simulink model "Activity_8"  (R2019b)
settings: Solver=VariableStepAuto  StartTime=0.0  StopTime=0.002  RelTol=1e-3
libraries: dspsrcs4 x3, dspfdesign x1
settings Model: Creator=linesLK  LastModifiedBy=linesLK

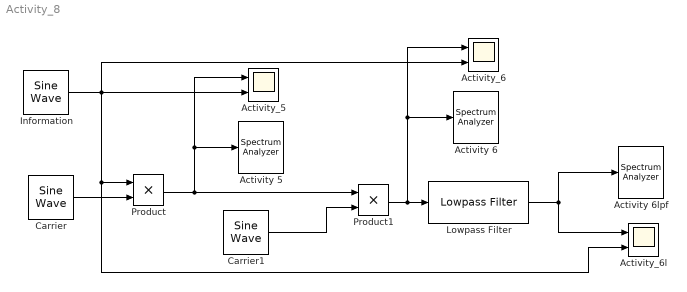
== system Activity_8 ==
  Activity 5 : SpectrumAnalyzer
  Activity 6 : SpectrumAnalyzer
  Activity 6lpf : SpectrumAnalyzer
  Activity_5 : Scope  NumInputPorts=2
  Activity_6 : Scope  NumInputPorts=2
  Activity_6l : Scope  NumInputPorts=2
  Carrier : dspsrcs4/Sine Wave  Amplitude=1  Frequency=15000  Phase=pi/2  SampleMode=Discrete  OutComplex=Real  CompMethod=Trigonometric fcn  TableSize=Speed  SampleTime=1/120000  SamplesPerFrame=1  ResetState=Restart at time zero  OutputFrames=off  dataType=double  wordLen=16  udDataType=sfix(16)  fracBitsMode=Best precision  numFracBits=15  OutDataTypeStr=double  LastOutDataTypeStr=double
  Carrier1 : dspsrcs4/Sine Wave  Amplitude=1  Frequency=15000  Phase=pi/2  SampleMode=Discrete  OutComplex=Real  CompMethod=Trigonometric fcn  TableSize=Speed  SampleTime=1/120000  SamplesPerFrame=1  ResetState=Restart at time zero  OutputFrames=off  dataType=double  wordLen=16  udDataType=sfix(16)  fracBitsMode=Best precision  numFracBits=15  OutDataTypeStr=double  LastOutDataTypeStr=double
  Information : dspsrcs4/Sine Wave  Amplitude=1  Frequency=1000  Phase=pi/2  SampleMode=Discrete  OutComplex=Real  CompMethod=Trigonometric fcn  TableSize=Speed  SampleTime=1/120000  SamplesPerFrame=1  ResetState=Restart at time zero  OutputFrames=off  dataType=double  wordLen=16  udDataType=sfix(16)  fracBitsMode=Best precision  numFracBits=15  OutDataTypeStr=double  LastOutDataTypeStr=double
  Lowpass Filter : dspfdesign/Lowpass Filter  FilterType=FIR  DesignForMinimumOrder=on  FilterOrder=50  PassbandFrequency=2e3  StopbandFrequency=10e3  PassbandRipple=0.1  StopbandAttenuation=80  InheritSampleRate=on  SampleRate=44100  SimulateUsing=Interpreted execution  roundingMode=Floor  coeffsDataTypeStr=fixdt(1,16)
  Product : Product
  Product1 : Product
  wires:
  Information/1 -> Activity_6/2, Activity_5/2, Activity_6l/2, Product/1
  Carrier/1 -> Product/2
  Product/1 -> Activity_5/1, Activity 5/1, Product1/1
  Carrier1/1 -> Product1/2
  Product1/1 -> Activity_6/1, Activity 6/1, Lowpass Filter/1
  Lowpass Filter/1 -> Activity_6l/1, Activity 6lpf/1
